simulink model "Aufgabe_1"  (R2012b)
settings: Solver=ode45  StartTime=0.0  StopTime=40.0  RelTol=1e-9
values from neighbouring files (symbols this model uses):
  c = 1    [init_A1.m]
  d = 1    [init_A1.m]
  m = 1    [init_A1.m]
settings Model: Creator=stschmid  LastModifiedBy=stschmid

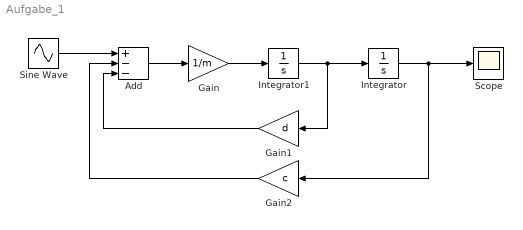
== system Aufgabe_1 ==
  Add : Sum  Inputs=+--
  Gain : Gain  Gain=1/m
  Gain1 : Gain  Gain=d
  Gain2 : Gain  Gain=c
  Integrator : Integrator
  Integrator1 : Integrator
  Scope : Scope
  Sine Wave : Sin  Frequency=10  SampleTime=0
  wires:
  Integrator1/1 -> Gain1/1, Integrator/1
  Integrator/1 -> Scope/1, Gain2/1
  Gain/1 -> Integrator1/1
  Add/1 -> Gain/1
  Gain1/1 -> Add/3
  Gain2/1 -> Add/2
  Sine Wave/1 -> Add/1
